simulink library "csci_fsw_mtv_lib"  (R2014b)
settings: Solver=ode45  StartTime=0.0  StopTime=10.0  RelTol=1e-3
libraries: util_info_lib x1, csc_act_actuator_manager_mtv_lib x1, csc_cmp_command_mode_process_mtv_lib x1, csc_cnt_attitude_control_lib_mtv x1, csc_egc_earth_grv_cancel_lib x1, csc_est_state_est_mtv_lib x1, csc_gdn_guidance_mtv_lib x1, csc_hio_hardware_io_mv_lib x1, csc_lc_limit_check_lib x1, csc_pcs_power_control_system_lib x1, csc_sc_wsim_stored_command_lib x1, csc_tcs_thermal_control_system_lib x1
settings Model: Creator=jkaidy  LastModifiedBy=tgorton

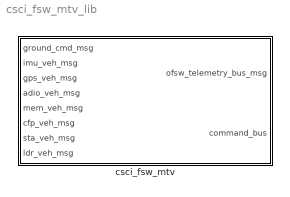
== system csci_fsw_mtv_lib ==
  csci_fsw_mtv : Subsystem

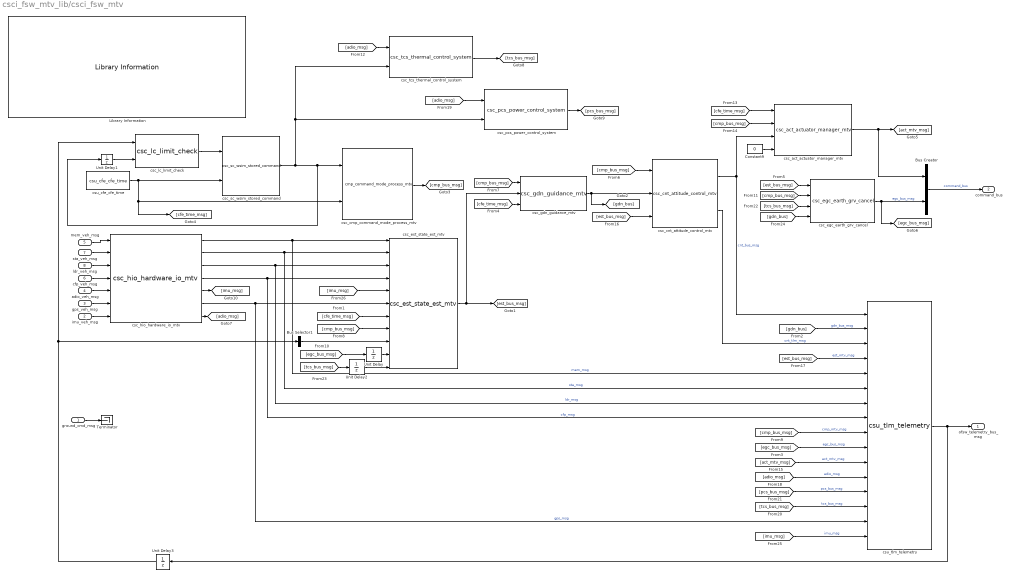
== system csci_fsw_mtv_lib/csci_fsw_mtv ==
  ground_cmd_msg : Inport
  imu_veh_msg : Inport  Port=2
  gps_veh_msg : Inport  Port=3
  adio_veh_msg : Inport  Port=4
  mem_veh_msg : Inport  Port=5
  cfp_veh_msg : Inport  Port=6
  sta_veh_msg : Inport  Port=7
  ldr_veh_msg : Inport  Port=8
  Bus Creator : BusCreator  Inputs=2
  Bus Selector1 : BusSelector  OutputSignals=act_mtv_msg  OutputAsBus=on
  Constant9 : Constant  Value=0  OutDataTypeStr=uint32
  Library Information : util_info_lib/Library Information  owner='NONE'
  Terminator : Terminator
  Unit Delay{,1..3} (4 alike) : UnitDelay  SampleTime=-1
  csc_act_actuator_manager_mtv : csc_act_actuator_manager_mtv_lib/csc_act_actuator_manager_mtv  Tag=OFSW; MDL_TICK=CNT_BUS_MSG
  csc_cmp_command_mode_process_mtv : csc_cmp_command_mode_process_mtv_lib/cmp_command_mode_process_mtv  Tag=OFSW
  csc_cnt_attitude_control_mtv : csc_cnt_attitude_control_lib_mtv/csc_cnt_attitude_control_mtv  Tag=OFSW; MDL_TICK=GDN_BUS_MSG
  csc_egc_earth_grv_cancel : csc_egc_earth_grv_cancel_lib/csc_egc_earth_grv_cancel  Tag=OFSW; MDL_TICK=TCS_BUS_MSG
  csc_est_state_est_mtv : csc_est_state_est_mtv_lib/csc_est_state_est_mtv  Tag=OFSW; MDL_TICK=CMP_MTV_MSG
  csc_gdn_guidance_mtv : csc_gdn_guidance_mtv_lib/csc_gdn_guidance_mtv  Tag=OFSW; MDL_TICK=EST_BUS_MSG
  csc_hio_hardware_io_mtv : csc_hio_hardware_io_mv_lib/csc_hio_hardware_io_mtv
  csc_lc_limit_check : csc_lc_limit_check_lib/csc_lc_limit_check
  csc_pcs_power_control_system : csc_pcs_power_control_system_lib/csc_pcs_power_control_system  Tag=OFSW; MDL_TICK=ADIO_MSG
  csc_sc_wsim_stored_command : csc_sc_wsim_stored_command_lib/csc_sc_wsim_stored_command
  csc_tcs_thermal_control_system : csc_tcs_thermal_control_system_lib/csc_tcs_thermal_control_system  Tag=OFSW; MDL_TICK=ADIO_MSG
  csu_cfe_cfe_time : csu_cfe_cfe_time_lib/csu_cfe_cfe_time  sch_dt=fsw_dt
  csu_tlm_telemetry : csu_tlm_telemetry_lib/csu_tlm_telemetry  num_inputs=16  output_bus_name=ofsw_telemetry_bus_msg
  ofsw_telemetry_bus_msg : Outport
  command_bus : Outport  Port=2
  wires:
  [imu_msg] -> csc_est_state_est_mtv/5
  [imu_msg] -> csu_tlm_telemetry/16  "imu_msg"
  csc_hio_hardware_io_mtv/5 -> [imu_msg]
  imu_veh_msg/1 -> csc_hio_hardware_io_mtv/7
  [gdn_bus] -> csc_egc_earth_grv_cancel/4
  Unit Delay2/1 -> csc_est_state_est_mtv/11
  [tcs_bus_msg] -> Unit Delay2/1
  csc_hio_hardware_io_mtv/6 -> csc_est_state_est_mtv/6, csu_tlm_telemetry/15  "gps_msg"
  gps_veh_msg/1 -> csc_hio_hardware_io_mtv/6
  [tcs_bus_msg] -> csc_egc_earth_grv_cancel/3
  [tcs_bus_msg] -> csu_tlm_telemetry/14  "tcs_bus_msg"
  [pcs_bus_msg] -> csu_tlm_telemetry/13  "pcs_bus_msg"
  csc_pcs_power_control_system/1 -> [pcs_bus_msg]
  csc_tcs_thermal_control_system/1 -> [tcs_bus_msg]
  [adio_msg] -> csc_pcs_power_control_system/1
  [adio_msg] -> csc_tcs_thermal_control_system/1
  [adio_msg] -> csu_tlm_telemetry/12  "adio_msg"
  csc_hio_hardware_io_mtv/7 -> [adio_msg]
  adio_veh_msg/1 -> csc_hio_hardware_io_mtv/5
  [cmp_bus_msg] -> csc_egc_earth_grv_cancel/2
  [est_bus_msg] -> csu_tlm_telemetry/4  "est_mtv_msg"
  [est_bus_msg] -> csc_cnt_attitude_control_mtv/3
  csc_hio_hardware_io_mtv/1 -> csc_est_state_est_mtv/1, csu_tlm_telemetry/5  "mem_msg"
  mem_veh_msg/1 -> csc_hio_hardware_io_mtv/1
  [act_mtv_msg] -> csu_tlm_telemetry/11  "act_mtv_msg"
  Constant9/1 -> csc_act_actuator_manager_mtv/4
  [cmp_bus_msg] -> csc_act_actuator_manager_mtv/2
  [cfe_time_msg] -> csc_act_actuator_manager_mtv/1
  csc_act_actuator_manager_mtv/1 -> Bus Creator/1, [act_mtv_msg]
  [gdn_bus] -> csu_tlm_telemetry/2  "gdn_bus_msg"
  Unit Delay/1 -> csc_est_state_est_mtv/10
  Bus Selector1/1 -> csc_est_state_est_mtv/9
  [cmp_bus_msg] -> csc_est_state_est_mtv/8
  [cfe_time_msg] -> csc_est_state_est_mtv/7
  csc_sc_wsim_stored_command/1 -> csc_cmp_command_mode_process_mtv/1, Unit Delay1/1, csc_pcs_power_control_system/2, csc_tcs_thermal_control_system/2
  csc_est_state_est_mtv/1 -> csc_gdn_guidance_mtv/2, [est_bus_msg]
  csc_gdn_guidance_mtv/1 -> [gdn_bus], csc_cnt_attitude_control_mtv/2
  csc_cnt_attitude_control_mtv/1 -> csu_tlm_telemetry/1, csc_act_actuator_manager_mtv/3  "cnt_bus_msg"
  ground_cmd_msg/1 -> Terminator/1
  csu_tlm_telemetry/1 -> ofsw_telemetry_bus_msg/1, Unit Delay3/1
  Bus Creator/1 -> command_bus/1  "command_bus"
  [cfe_time_msg] -> csc_gdn_guidance_mtv/3
  csu_cfe_cfe_time/1 -> csc_sc_wsim_stored_command/2, [cfe_time_msg], csc_cmp_command_mode_process_mtv/2
  csc_cmp_command_mode_process_mtv/1 -> [cmp_bus_msg]
  [cmp_bus_msg] -> csc_cnt_attitude_control_mtv/1
  [cmp_bus_msg] -> csc_gdn_guidance_mtv/1
  csc_cnt_attitude_control_mtv/2 -> csu_tlm_telemetry/3  "cnt_tlm_msg"
  sta_veh_msg/1 -> csc_hio_hardware_io_mtv/2
  ldr_veh_msg/1 -> csc_hio_hardware_io_mtv/3
  cfp_veh_msg/1 -> csc_hio_hardware_io_mtv/4
  csc_hio_hardware_io_mtv/2 -> csc_est_state_est_mtv/2, csu_tlm_telemetry/6  "sta_msg"
  csc_hio_hardware_io_mtv/3 -> csc_est_state_est_mtv/3, csu_tlm_telemetry/7  "ldr_msg"
  csc_hio_hardware_io_mtv/4 -> csc_est_state_est_mtv/4, csu_tlm_telemetry/8  "cfp_msg"
  [cmp_bus_msg] -> csu_tlm_telemetry/9  "cmp_mtv_msg"
  csc_lc_limit_check/1 -> csc_sc_wsim_stored_command/1
  Unit Delay3/1 -> Bus Selector1/1, csc_lc_limit_check/1
  Unit Delay1/1 -> csc_lc_limit_check/2
  [est_bus_msg] -> csc_egc_earth_grv_cancel/1
  csc_egc_earth_grv_cancel/1 -> [egc_bus_msg], Bus Creator/2  "egc_bus_msg"
  [egc_bus_msg] -> csu_tlm_telemetry/10  "egc_bus_msg"
  [egc_bus_msg] -> Unit Delay/1
